simulink model "Frequency_Mixer"  (R2014b)
settings: Solver=ode3  StartTime=0.0  StopTime=1  FixedStep=1/5000000  RelTol=1e-3
libraries: commsynccomp2 x1, simulink x1
settings Model: Creator=Eitima  LastModifiedBy=Eitima
settings DataIOCC: ExternalInput=[t, SigTime]  LimitDataPoints=off  LoadExternalInput=on  TimeSaveName=tOut  OutputSaveName=SigTimeOut

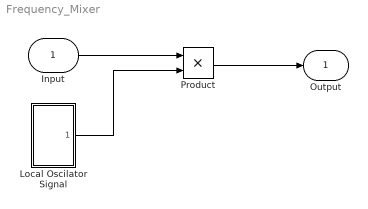
== system Frequency_Mixer ==
  Input : Inport
  Local Oscilator Signal : Subsystem
  Product : Product
  Output : Outport
  wires:
  Input/1 -> Product/1
  Local Oscilator Signal/1(Output) -> Product/2
  Product/1 -> Output/1

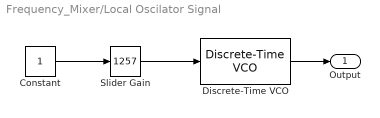
== system Frequency_Mixer/Local Oscilator Signal ==
  Constant : Constant
  Discrete-Time VCO : commsynccomp2/Discrete-Time VCO  Ac=1  Fc=0  Kc=1000  Ph=0  ts=1/5000000
  Slider Gain : simulink/Math Operations/Slider Gain  low=1015  gain=1257  high=2070
  Output : Outport
  wires:
  Constant/1 -> Slider Gain/1
  Slider Gain/1 -> Discrete-Time VCO/1
  Discrete-Time VCO/1 -> Output/1
